simulink library "asbhl20RF"  (R2016b)
settings: Solver=VariableStepAuto  StartTime=0.0  StopTime=10.0  RelTol=1e-3
undefined symbols (not defined in the file): Ts
Description:
  | HL-20 communications signal access component module (stub)
  | 
  | Copyright 1990-2005 The MathWorks Inc.
settings Model: Creator=The MathWorks, Inc.  LastModifiedBy=The MathWorks, Inc.
settings DataIOCC: SaveFormat=Array  SignalLoggingSaveFormat=ModelDataLogs
settings OptimizationCC: BlockReduction=off  BooleanDataType=off
settings DebuggingCC: SaveWithParameterizedLinksMsg=none  UnderspecifiedInitializationDetection=Classic  MergeDetectMultiDrivingBlocksExec=none  SignalResolutionControl=TryResolveAllWithWarning  MultiTaskCondExecSysMsg=none  StrictBusMsg=None
settings HardwareCC: ProdBitPerPointer=32  ProdBitPerSizeT=32  ProdBitPerPtrDiffT=32  ProdLargestAtomicFloat=None  ProdIntDivRoundTo=Undefined  ProdEndianess=Unspecified  ProdWordSize=32  ProdHWDeviceType=32-bit Generic  TargetUnknown=on
settings ModelReferenceCC: PropagateSignalLabelsOutOfModel=off
settings ConfigComp: CovMetricSettings=dw  CovHtmlReporting=on  CovSaveCumulativeToWorkspaceVar=on  CovSaveSingleToWorkspaceVar=on  CovExternalEMLEnable=off

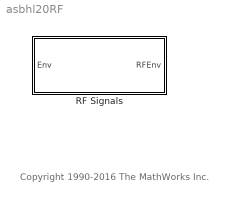
== system asbhl20RF ==
  note: Copyright 1990-2016 The MathWorks Inc.
  RF Signals : Subsystem  TreatAsAtomicUnit=on

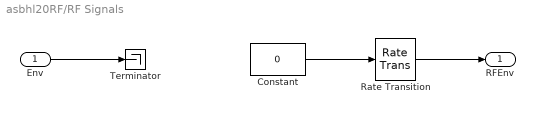
== system asbhl20RF/RF Signals ==
  Env : Inport
  Constant : Constant  Value=0  SampleTime=Ts
  Rate Transition : RateTransition  OutPortSampleTime=0
  Terminator : Terminator
  RFEnv : Outport
  wires:
  Rate Transition/1 -> RFEnv/1
  Constant/1 -> Rate Transition/1
  Env/1 -> Terminator/1
